simulink library "Arrowhead_Lib"  (R2026a)
settings: Solver=VariableStepAuto
undefined symbols (not defined in the file): X, Y, Z
libraries: sm_lib x17, $bdroot x3, nesl_utility x2, fl_lib x1
Description:
  | Copyright 2022-2026 The MathWorks, Inc.
settings Model: Creator=smiller  LastModifiedBy=smiller

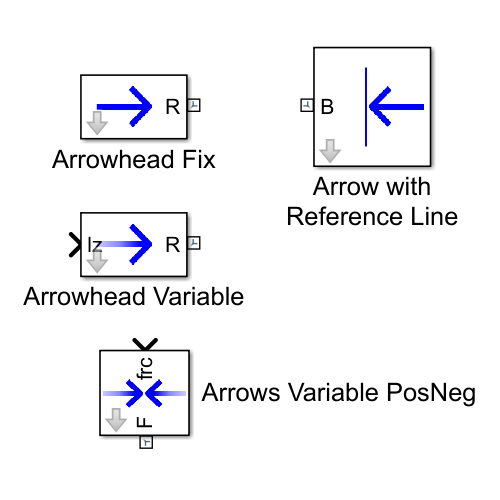
[thumbnail: Simulink's stored preview of the top-level diagram]
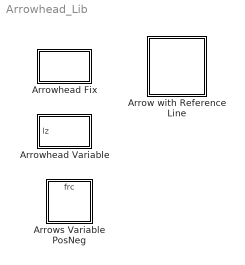
== system Arrowhead_Lib ==
  Arrow with Reference Line : Subsystem  mask{tip_l=1, tip_a=90, shaft_len=2, line_width=0.2, arrow_opc=0.5, arrow_depth=0.5, arrow_clr=[1.0 0.6 0.0], ref_ax_opc=0.5, ref_ax_offset=0.125, ref_ax_dim=[4 0.06 0.04], ref_ax_clr=[1.0 0.6 0.0]}
      mask prompts: tip_l "Tip Length (m)"; tip_a "Tip Angle (deg)"; shaft_len "Shaft Length (m)"; line_width "Line Width (m)"; arrow_opc "Arrow Opacity (0-1)"; arrow_depth "Arrow Depth (m)"; arrow_clr "Color Arrow [RGB] (0-1)"; ref_ax_opc "Opacity (0-1)"; ref_ax_offset "Offset along x (% of x length)"; ref_ax_dim "Dimensions (m)"; ref_ax_clr "Color [RGB] (0-1)"
      mask TypeOptions tip_l: Arrow/tip_l
      mask TypeOptions tip_a: Arrow/tip_a
      mask TypeOptions shaft_len: Arrow/shaft_len
      mask TypeOptions line_width: Arrow/line_width
      mask TypeOptions arrow_opc: Arrow/arrow_opc
      mask TypeOptions arrow_depth: Arrow/arrow_depth
      mask TypeOptions arrow_clr: Arrow/arrow_clr
      mask TypeOptions ref_ax_opc:
      | Reference
      | Axis/ref_ax_opc
      mask TypeOptions ref_ax_offset:
      | Reference
      | Axis/ref_ax_offset
      mask TypeOptions ref_ax_dim:
      | Reference
      | Axis/ref_ax_dim
      mask TypeOptions ref_ax_clr:
      | Reference
      | Axis/ref_ax_clr
      mask DialogControl Container4 Prompt: Arrow
      mask DialogControl Container3 Prompt: Reference Line
      mask Display: image('Arrow_with_Reference_Line_IMAGE.png')
  Arrowhead Fix : Subsystem  mask{shaft_len=2, tip_l=1, tip_a=90, arrow_clr=[0.3922 0.8314 0.07451], arrow_opc=1, arrow_depth=0.5, line_width=0.2}
      mask prompts: shaft_len "Shaft Length (m)"; tip_l "Tip Length (m)"; tip_a "Tip Angle (deg)"; arrow_clr "Color Arrow [RGB] (0-1)"; arrow_opc "Arrow Opacity (0-1)"; arrow_depth "Arrow Depth (m)"; line_width "Line Width (m)"
      mask Display: image('Arrowhead_Fix_IMAGE.png')
  Arrowhead Variable : Subsystem  mask{tip_l=1, tip_a=90, line_width=0.2, arrow_depth=0.5, arrow_clr=[0.3922 0.8314 0.07451], arrow_opc=1}
      mask prompts: tip_l "Tip Length (m)"; tip_a "Tip Angle (deg)"; line_width "Line Width (m)"; arrow_depth "Line Depth (m)"; arrow_clr "Arrow Color [RGB] (0-1)"; arrow_opc "Arrow Opacity (0-1)"
      mask Display: image('Arrowhead_Variable_IMAGE.png')
  Arrows Variable PosNeg : Subsystem  mask{max_force=4e5, max_length=10, arrow_clr=[0.3922 0.8314 0.07451], arrow_depth=0.5, line_width=0.2, tip_a=90, tip_l=1, arrow_opc=0.5}
      mask prompts: max_force "Max Force (N)"; max_length "Max Length (m)"; arrow_clr "Color Arrow [RGB] (0-1)"; arrow_depth "Arrow Depth (m)"; line_width "Line Width (m)"; tip_a "Tip Angle (deg)"; tip_l "Tip Length (m)"; arrow_opc "Arrow Opacity (0-1)"
      mask TypeOptions arrow_clr: Arrowhead Neg/arrow_clr | Arrowhead Pos/arrow_clr
      mask TypeOptions arrow_depth: Arrowhead Neg/arrow_depth | Arrowhead Pos/arrow_depth
      mask TypeOptions line_width: Arrowhead Neg/line_width | Arrowhead Pos/line_width
      mask TypeOptions tip_a: Arrowhead Neg/tip_a | Arrowhead Pos/tip_a
      mask TypeOptions tip_l: Arrowhead Neg/tip_l | Arrowhead Pos/tip_l
      mask TypeOptions arrow_opc: Arrowhead Neg/arrow_opc | Arrowhead Pos/arrow_opc
      mask Display: image('Arrows_Variable_PosNeg_IMAGE.png')

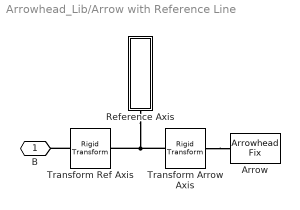
== system Arrowhead_Lib/Arrow with Reference Line ==
  Arrow : $bdroot/Arrowhead Fix  shaft_len=shaft_len  tip_l=tip_l  tip_a=tip_a  arrow_clr=arrow_clr  arrow_opc=arrow_opc  arrow_depth=arrow_depth  line_width=line_width
  Reference Axis : Subsystem  mask{ref_ax_dim=ref_ax_dim, ref_ax_offset=ref_ax_offset, ref_ax_clr=ref_ax_clr, ref_ax_opc=ref_ax_opc}
      mask prompts: ref_ax_dim "Dimensions (m)"; ref_ax_offset "Offset along x (% of x length)"; ref_ax_clr "Color [RGB] (0-1)"; ref_ax_opc "Opacity (0-1)"
  Transform Arrow Axis : sm_lib/Frames and Transforms/Rigid Transform  RotationMethod=RotationSequence  FollAlignAxisA=+X  BaseAlignAxisA=+Y  FollAlignAxisB=+Y  BaseAlignAxisB=+Z  RotationStandardAxis=+X  RotationAngle=-90  RotationAngleUnits=deg  RotationArbitraryAxis=[0 0 1]  RotationSequenceAxes=FollowerAxes  RotationSequence=XYZ  RotationSequenceAngles=[90 0 90]  RotationSequenceAnglesUnits=deg  RotationMatrix=[1 0 0; 0 1 0; 0 0 1]  Quaternion=[1 0 0 0]  TranslationMethod=None  TranslationCartesianOffset=[0 0 0]  TranslationCartesianOffsetUnits=m  TranslationStandardAxis=+Z  TranslationStandardOffset=0  TranslationStandardOffsetUnits=m  TranslationROffset=0  TranslationROffsetUnits=m  TranslationThetaOffset=0  TranslationThetaOffsetUnits=deg  TranslationZOffset=0  TranslationZOffsetUnits=m
  Transform Ref Axis : sm_lib/Frames and Transforms/Rigid Transform  RotationMethod=StandardAxis  FollAlignAxisA=+X  BaseAlignAxisA=+Y  FollAlignAxisB=+Y  BaseAlignAxisB=+Z  RotationStandardAxis=+Z  RotationAngle=90  RotationAngleUnits=deg  RotationArbitraryAxis=[0 0 1]  RotationSequenceAxes=FollowerAxes  RotationSequence=XYZ  RotationSequenceAngles=[90 0 90]  RotationSequenceAnglesUnits=deg  RotationMatrix=[1 0 0; 0 1 0; 0 0 1]  Quaternion=[1 0 0 0]  TranslationMethod=None  TranslationCartesianOffset=[0 0 0]  TranslationCartesianOffsetUnits=m  TranslationStandardAxis=+Z  TranslationStandardOffset=0  TranslationStandardOffsetUnits=m  TranslationROffset=0  TranslationROffsetUnits=m  TranslationThetaOffset=0  TranslationThetaOffsetUnits=deg  TranslationZOffset=0  TranslationZOffsetUnits=m
  B : PMIOPort  Side=Left
  connections:
  Transform Arrow Axis/RConn1 -- Arrow/RConn1
  Transform Arrow Axis/LConn1 -- Reference Axis/LConn1 -- Transform Ref Axis/RConn1
  Transform Ref Axis/LConn1 -- B/RConn1

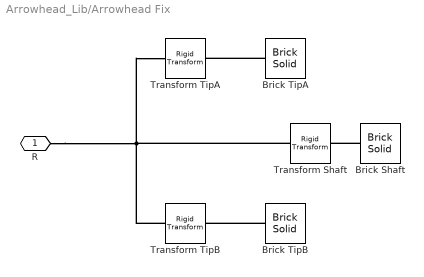
== system Arrowhead_Lib/Arrowhead Fix ==
  Brick Shaft : sm_lib/Body Elements/Brick Solid  BrickDimensions=[arrow_depth line_width shaft_len]  BrickDimensionsUnits=m  ExportEntireGeometry=off  InertiaType=PointMass  BasedOnType=Density  Density=1000  DensityUnits=kg/m^3  Mass=1e-3  MassUnits=kg  CenterOfMass=[0 0 0]  CenterOfMassUnits=m  MomentsOfInertia=[1 1 1]  MomentsOfInertiaUnits=kg*m^2  ProductsOfInertia=[0 0 0]  ProductsOfInertiaUnits=kg*m^2  GraphicType=FromGeometry  MarkerShape=Sphere  MarkerSize=10  GraphicVisPropType=AdvancedVisualProperties  GraphicDiffuseColor=[arrow_clr arrow_opc]  GraphicOpacity=1.0  GraphicSpecularColor=[0.5 0.5 0.5 arrow_opc]  GraphicAmbientColor=[0.15 0.15 0.15 arrow_opc]  GraphicEmissiveColor=[arrow_clr*0.3 arrow_opc]  GraphicShininess=75  DoExposeReferenceFrame=off  SerializedFrames=<Frames><Frame><Id>Frame1</Id><Value><Name>B</Name><Origin><Source>GeometricFeature</Source><FeatureName>-z surface</FeatureName></Origin><PrimaryAxis><DefinedDirection>+Z</DefinedDirection><Source>ReferenceFrame</Source><SourceDirection>+Z</SourceDirection><FeatureName></FeatureName></PrimaryAxis><SecondaryAxis><DefinedDirection>+X</DefinedDirection><Source>ReferenceFrame</Source><SourceDirection>+X</SourceDirection><FeatureName></FeatureName></SecondaryAxis></Value></Frame></Frames>
  Brick TipA : sm_lib/Body Elements/Brick Solid  BrickDimensions=[arrow_depth line_width tip_l]  BrickDimensionsUnits=m  ExportEntireGeometry=off  InertiaType=PointMass  BasedOnType=Mass  Density=1000  DensityUnits=kg/m^3  Mass=1e-3  MassUnits=kg  CenterOfMass=[0 0 0]  CenterOfMassUnits=m  MomentsOfInertia=[1 1 1]  MomentsOfInertiaUnits=kg*m^2  ProductsOfInertia=[0 0 0]  ProductsOfInertiaUnits=kg*m^2  GraphicType=FromGeometry  MarkerShape=Sphere  MarkerSize=10  GraphicVisPropType=AdvancedVisualProperties  GraphicDiffuseColor=[arrow_clr arrow_opc]  GraphicOpacity=1.0  GraphicSpecularColor=[0.5 0.5 0.5 arrow_opc]  GraphicAmbientColor=[0.15 0.15 0.15 arrow_opc]  GraphicEmissiveColor=[arrow_clr*0.3 arrow_opc]  GraphicShininess=75  DoExposeReferenceFrame=off  SerializedFrames=<Frames><Frame><Id>Frame1</Id><Value><Name>B</Name><Origin><Source>GeometricFeature</Source><FeatureName>-z surface</FeatureName></Origin><PrimaryAxis><DefinedDirection>+Z</DefinedDirection><Source>ReferenceFrame</Source><SourceDirection>+Z</SourceDirection><FeatureName></FeatureName></PrimaryAxis><SecondaryAxis><DefinedDirection>+X</DefinedDirection><Source>ReferenceFrame</Source><SourceDirection>+X</SourceDirection><FeatureName></FeatureName></SecondaryAxis></Value></Frame></Frames>
  Brick TipB : sm_lib/Body Elements/Brick Solid  BrickDimensions=[arrow_depth line_width tip_l]  BrickDimensionsUnits=m  ExportEntireGeometry=off  InertiaType=PointMass  BasedOnType=Density  Density=1000  DensityUnits=kg/m^3  Mass=1e-3  MassUnits=kg  CenterOfMass=[0 0 0]  CenterOfMassUnits=m  MomentsOfInertia=[1 1 1]  MomentsOfInertiaUnits=kg*m^2  ProductsOfInertia=[0 0 0]  ProductsOfInertiaUnits=kg*m^2  GraphicType=FromGeometry  MarkerShape=Sphere  MarkerSize=10  GraphicVisPropType=AdvancedVisualProperties  GraphicDiffuseColor=[arrow_clr arrow_opc]  GraphicOpacity=1.0  GraphicSpecularColor=[0.5 0.5 0.5 arrow_opc]  GraphicAmbientColor=[0.15 0.15 0.15 arrow_opc]  GraphicEmissiveColor=[arrow_clr*0.3 arrow_opc]  GraphicShininess=75  DoExposeReferenceFrame=off  SerializedFrames=<Frames><Frame><Id>Frame1</Id><Value><Name>B</Name><Origin><Source>GeometricFeature</Source><FeatureName>-z surface</FeatureName></Origin><PrimaryAxis><DefinedDirection>+Z</DefinedDirection><Source>ReferenceFrame</Source><SourceDirection>+Z</SourceDirection><FeatureName></FeatureName></PrimaryAxis><SecondaryAxis><DefinedDirection>+X</DefinedDirection><Source>ReferenceFrame</Source><SourceDirection>+X</SourceDirection><FeatureName></FeatureName></SecondaryAxis></Value></Frame></Frames>
  Transform Shaft : sm_lib/Frames and Transforms/Rigid Transform  RotationMethod=None  FollAlignAxisA=+X  BaseAlignAxisA=+Y  FollAlignAxisB=+Y  BaseAlignAxisB=+Z  RotationStandardAxis=+Z  RotationAngle=0.0  RotationAngleUnits=deg  RotationArbitraryAxis=[0 0 1]  RotationSequenceAxes=FollowerAxes  RotationSequence=XYX  RotationSequenceAngles=[0 0 0]  RotationSequenceAnglesUnits=deg  RotationMatrix=[1 0 0; 0 1 0; 0 0 1]  Quaternion=[1 0 0 0]  TranslationMethod=StandardAxis  TranslationCartesianOffset=[0 0 0]  TranslationCartesianOffsetUnits=m  TranslationStandardAxis=+Z  TranslationStandardOffset=(line_width/2)/tand(tip_a/2)  TranslationStandardOffsetUnits=m  TranslationROffset=0  TranslationROffsetUnits=m  TranslationThetaOffset=0  TranslationThetaOffsetUnits=deg  TranslationZOffset=0  TranslationZOffsetUnits=m
  Transform TipA : sm_lib/Frames and Transforms/Rigid Transform  RotationMethod=StandardAxis  FollAlignAxisA=+X  BaseAlignAxisA=+Y  FollAlignAxisB=+Y  BaseAlignAxisB=+Z  RotationStandardAxis=+X  RotationAngle=tip_a/2  RotationAngleUnits=deg  RotationArbitraryAxis=[0 0 1]  RotationSequenceAxes=FollowerAxes  RotationSequence=XYX  RotationSequenceAngles=[0 0 0]  RotationSequenceAnglesUnits=deg  RotationMatrix=[1 0 0; 0 1 0; 0 0 1]  Quaternion=[1 0 0 0]  TranslationMethod=Cartesian  TranslationCartesianOffset=[0 0 0]*tip_l/2*sind(tip_a/2)+[0 1 1]*line_width/2*sind(tip_a/2)  TranslationCartesianOffsetUnits=m  TranslationStandardAxis=+Y  TranslationStandardOffset=tip_l/2*sind(tip_a/2)  TranslationStandardOffsetUnits=m  TranslationROffset=0  TranslationROffsetUnits=m  TranslationThetaOffset=0  TranslationThetaOffsetUnits=deg  TranslationZOffset=0  TranslationZOffsetUnits=m
  Transform TipB : sm_lib/Frames and Transforms/Rigid Transform  RotationMethod=StandardAxis  FollAlignAxisA=+X  BaseAlignAxisA=+Y  FollAlignAxisB=+Y  BaseAlignAxisB=+Z  RotationStandardAxis=-X  RotationAngle=tip_a/2  RotationAngleUnits=deg  RotationArbitraryAxis=[0 0 1]  RotationSequenceAxes=FollowerAxes  RotationSequence=XYX  RotationSequenceAngles=[0 0 0]  RotationSequenceAnglesUnits=deg  RotationMatrix=[1 0 0; 0 1 0; 0 0 1]  Quaternion=[1 0 0 0]  TranslationMethod=Cartesian  TranslationCartesianOffset=[0 0 0]*tip_l/2*sind(tip_a/2)+[0 -1 1]*line_width/2*sind(tip_a/2)  TranslationCartesianOffsetUnits=m  TranslationStandardAxis=+Y  TranslationStandardOffset=tip_l/2*sind(tip_a/2)  TranslationStandardOffsetUnits=m  TranslationROffset=0  TranslationROffsetUnits=m  TranslationThetaOffset=0  TranslationThetaOffsetUnits=deg  TranslationZOffset=0  TranslationZOffsetUnits=m
  R : PMIOPort  Side=Right
  connections:
  Brick Shaft/LConn1 -- Transform Shaft/RConn1
  Brick TipB/LConn1 -- Transform TipB/RConn1
  Transform TipB/LConn1 -- Transform Shaft/LConn1 -- Transform TipA/LConn1 -- R/RConn1
  Brick TipA/LConn1 -- Transform TipA/RConn1

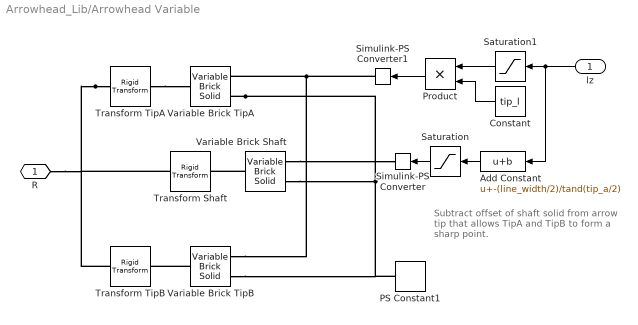
== system Arrowhead_Lib/Arrowhead Variable ==
  note: Subtract offset of shaft solid from arrow tip that allows TipA and TipB to form a sharp point.
  lz : Inport
  Add Constant : Bias  Bias=-(line_width/2)/tand(tip_a/2)  SaturateOnIntegerOverflow=off
  Constant : Constant  Value=tip_l
  PS Constant1 : fl_lib/Physical Signals/Sources/PS Constant  constant=1e-3 kg
  Product : Product
  Saturation : Saturate  UpperLimit=Inf  LowerLimit=1e-3  ZeroCross=off
  Saturation1 : Saturate  UpperLimit=1  LowerLimit=1e-3  ZeroCross=off
  Simulink-PS Converter : nesl_utility/Simulink-PS Converter  PhysicalDomain=network_engine_domain  SubClassName=ps_input  LeftPortType=input  RightPortType=output  PseudoPeriodic=off  Frequencies=[]  NoiseDistribution=none  NoiseParameters=[]  Unit=1  AffineConversion=off  FilteringAndDerivatives=provide  SimscapeFilterOrder=1  InputFilterTimeConstant=0.001  UdotUserProvided=0
  Simulink-PS Converter1 : nesl_utility/Simulink-PS Converter  PhysicalDomain=network_engine_domain  SubClassName=ps_input  LeftPortType=input  RightPortType=output  PseudoPeriodic=off  Frequencies=[]  NoiseDistribution=none  NoiseParameters=[]  Unit=1  AffineConversion=off  FilteringAndDerivatives=provide  SimscapeFilterOrder=1  InputFilterTimeConstant=0.001  UdotUserProvided=0
  Transform Shaft : sm_lib/Frames and Transforms/Rigid Transform  RotationMethod=None  FollAlignAxisA=+X  BaseAlignAxisA=+Y  FollAlignAxisB=+Y  BaseAlignAxisB=+Z  RotationStandardAxis=+Z  RotationAngle=0.0  RotationAngleUnits=deg  RotationArbitraryAxis=[0 0 1]  RotationSequenceAxes=FollowerAxes  RotationSequence=XYX  RotationSequenceAngles=[0 0 0]  RotationSequenceAnglesUnits=deg  RotationMatrix=[1 0 0; 0 1 0; 0 0 1]  Quaternion=[1 0 0 0]  TranslationMethod=StandardAxis  TranslationCartesianOffset=[0 0 0]  TranslationCartesianOffsetUnits=m  TranslationStandardAxis=+Z  TranslationStandardOffset=(line_width/2)/tand(tip_a/2)  TranslationStandardOffsetUnits=m  TranslationROffset=0  TranslationROffsetUnits=m  TranslationThetaOffset=0  TranslationThetaOffsetUnits=deg  TranslationZOffset=0  TranslationZOffsetUnits=m
  Transform TipA : sm_lib/Frames and Transforms/Rigid Transform  RotationMethod=StandardAxis  FollAlignAxisA=+X  BaseAlignAxisA=+Y  FollAlignAxisB=+Y  BaseAlignAxisB=+Z  RotationStandardAxis=+X  RotationAngle=tip_a/2  RotationAngleUnits=deg  RotationArbitraryAxis=[0 0 1]  RotationSequenceAxes=FollowerAxes  RotationSequence=XYX  RotationSequenceAngles=[0 0 0]  RotationSequenceAnglesUnits=deg  RotationMatrix=[1 0 0; 0 1 0; 0 0 1]  Quaternion=[1 0 0 0]  TranslationMethod=Cartesian  TranslationCartesianOffset=[0 0 0]*tip_l/2*sind(tip_a/2)+[0 1 1]*line_width/2*sind(tip_a/2)  TranslationCartesianOffsetUnits=m  TranslationStandardAxis=+Y  TranslationStandardOffset=tip_l/2*sind(tip_a/2)  TranslationStandardOffsetUnits=m  TranslationROffset=0  TranslationROffsetUnits=m  TranslationThetaOffset=0  TranslationThetaOffsetUnits=deg  TranslationZOffset=0  TranslationZOffsetUnits=m
  Transform TipB : sm_lib/Frames and Transforms/Rigid Transform  RotationMethod=StandardAxis  FollAlignAxisA=+X  BaseAlignAxisA=+Y  FollAlignAxisB=+Y  BaseAlignAxisB=+Z  RotationStandardAxis=-X  RotationAngle=tip_a/2  RotationAngleUnits=deg  RotationArbitraryAxis=[0 0 1]  RotationSequenceAxes=FollowerAxes  RotationSequence=XYX  RotationSequenceAngles=[0 0 0]  RotationSequenceAnglesUnits=deg  RotationMatrix=[1 0 0; 0 1 0; 0 0 1]  Quaternion=[1 0 0 0]  TranslationMethod=Cartesian  TranslationCartesianOffset=[0 0 0]*tip_l/2*sind(tip_a/2)+[0 -1 1]*line_width/2*sind(tip_a/2)  TranslationCartesianOffsetUnits=m  TranslationStandardAxis=+Y  TranslationStandardOffset=tip_l/2*sind(tip_a/2)  TranslationStandardOffsetUnits=m  TranslationROffset=0  TranslationROffsetUnits=m  TranslationThetaOffset=0  TranslationThetaOffsetUnits=deg  TranslationZOffset=0  TranslationZOffsetUnits=m
  Variable Brick Shaft : sm_lib/Body Elements/Variable Mass/Variable Brick Solid  ComputedVariable=Density  XLengthType=Constant  XLength=arrow_depth  XLengthUnits=m  YLengthType=Constant  YLength=line_width  YLengthUnits=m  ZLengthType=ProvidedByInput  ZLength=0.5  ZLengthUnits=m  DensityType=Constant  Density=1000  DensityUnits=kg/m^3  MassType=ProvidedByInput  Mass=1  MassUnits=kg  SenseXLength=off  SenseYLength=off  SenseZLength=off  SenseDensity=off  SenseMass=off  SenseCenterOfMass=off  SenseInertiaMatrix=off  GraphicType=FromGeometry  MarkerShape=Sphere  MarkerSize=10  GraphicVisPropType=AdvancedVisualProperties  GraphicDiffuseColor=[arrow_clr arrow_opc]  GraphicOpacity=1.0  GraphicSpecularColor=[0.5 0.5 0.5 arrow_opc]  GraphicAmbientColor=[0.15 0.15 0.15 arrow_opc]  GraphicEmissiveColor=[arrow_clr*0.3 arrow_opc]  GraphicShininess=75
  Variable Brick TipA : sm_lib/Body Elements/Variable Mass/Variable Brick Solid  ComputedVariable=Density  XLengthType=Constant  XLength=arrow_depth  XLengthUnits=m  YLengthType=Constant  YLength=line_width  YLengthUnits=m  ZLengthType=ProvidedByInput  ZLength=0.5  ZLengthUnits=m  DensityType=Constant  Density=1000  DensityUnits=kg/m^3  MassType=ProvidedByInput  Mass=1  MassUnits=kg  SenseXLength=off  SenseYLength=off  SenseZLength=off  SenseDensity=off  SenseMass=off  SenseCenterOfMass=off  SenseInertiaMatrix=off  GraphicType=FromGeometry  MarkerShape=Sphere  MarkerSize=10  GraphicVisPropType=AdvancedVisualProperties  GraphicDiffuseColor=[arrow_clr arrow_opc]  GraphicOpacity=1.0  GraphicSpecularColor=[0.5 0.5 0.5 arrow_opc]  GraphicAmbientColor=[0.15 0.15 0.15 arrow_opc]  GraphicEmissiveColor=[arrow_clr*0.3 arrow_opc]  GraphicShininess=75
  Variable Brick TipB : sm_lib/Body Elements/Variable Mass/Variable Brick Solid  ComputedVariable=Density  XLengthType=Constant  XLength=arrow_depth  XLengthUnits=m  YLengthType=Constant  YLength=line_width  YLengthUnits=m  ZLengthType=ProvidedByInput  ZLength=0.5  ZLengthUnits=m  DensityType=Constant  Density=1000  DensityUnits=kg/m^3  MassType=ProvidedByInput  Mass=1  MassUnits=kg  SenseXLength=off  SenseYLength=off  SenseZLength=off  SenseDensity=off  SenseMass=off  SenseCenterOfMass=off  SenseInertiaMatrix=off  GraphicType=FromGeometry  MarkerShape=Sphere  MarkerSize=10  GraphicVisPropType=AdvancedVisualProperties  GraphicDiffuseColor=[arrow_clr arrow_opc]  GraphicOpacity=1.0  GraphicSpecularColor=[0.5 0.5 0.5 arrow_opc]  GraphicAmbientColor=[0.15 0.15 0.15 arrow_opc]  GraphicEmissiveColor=[arrow_clr*0.3 arrow_opc]  GraphicShininess=75
  R : PMIOPort  Side=Right
  wires:
  lz/1 -> Add Constant/1, Saturation1/1
  Saturation/1 -> Simulink-PS Converter/1
  Saturation1/1 -> Product/1
  Constant/1 -> Product/2
  Product/1 -> Simulink-PS Converter1/1
  Add Constant/1 -> Saturation/1
  connections:
  Variable Brick Shaft/RConn1 -- Transform Shaft/RConn1
  Variable Brick TipB/RConn1 -- Transform TipB/RConn1
  Transform TipA/LConn1 -- R/RConn1 -- Transform TipB/LConn1 -- Transform Shaft/LConn1
  Variable Brick TipA/LConn2 -- Variable Brick Shaft/LConn2 -- Variable Brick TipB/LConn2 -- PS Constant1/RConn1
  Transform TipA/RConn1 -- Variable Brick TipA/RConn1
  Simulink-PS Converter1/RConn1 -- Variable Brick TipB/LConn1 -- Variable Brick TipA/LConn1
  Variable Brick Shaft/LConn1 -- Simulink-PS Converter/RConn1

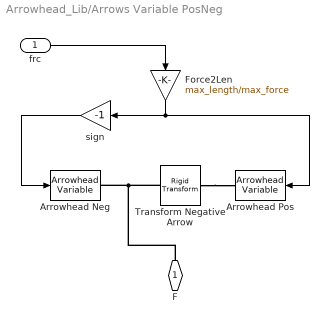
== system Arrowhead_Lib/Arrows Variable PosNeg ==
  frc : Inport
  Arrowhead Neg : $bdroot/Arrowhead Variable  tip_l=tip_l  tip_a=tip_a  line_width=line_width  arrow_depth=arrow_depth  arrow_clr=arrow_clr  arrow_opc=arrow_opc
  Arrowhead Pos : $bdroot/Arrowhead Variable  tip_l=tip_l  tip_a=tip_a  line_width=line_width  arrow_depth=arrow_depth  arrow_clr=arrow_clr  arrow_opc=arrow_opc
  Force2Len : Gain  Gain=max_length/max_force
  Transform Negative Arrow : sm_lib/Frames and Transforms/Rigid Transform  RotationMethod=StandardAxis  FollAlignAxisA=+X  BaseAlignAxisA=+Y  FollAlignAxisB=+Y  BaseAlignAxisB=+Z  RotationStandardAxis=+X  RotationAngle=180  RotationAngleUnits=deg  RotationArbitraryAxis=[0 0 1]  RotationSequenceAxes=FollowerAxes  RotationSequence=XYX  RotationSequenceAngles=[0 0 0]  RotationSequenceAnglesUnits=deg  RotationMatrix=[1 0 0; 0 1 0; 0 0 1]  Quaternion=[1 0 0 0]  TranslationMethod=None  TranslationCartesianOffset=[0 0 0]  TranslationCartesianOffsetUnits=m  TranslationStandardAxis=+Z  TranslationStandardOffset=0  TranslationStandardOffsetUnits=m  TranslationROffset=0  TranslationROffsetUnits=m  TranslationThetaOffset=0  TranslationThetaOffsetUnits=deg  TranslationZOffset=0  TranslationZOffsetUnits=m
  sign : Gain  Gain=-1
  F : PMIOPort  Side=Right
  wires:
  frc/1 -> Force2Len/1
  Force2Len/1 -> Arrowhead Pos/1, sign/1
  sign/1 -> Arrowhead Neg/1
  connections:
  Transform Negative Arrow/RConn1 -- Arrowhead Pos/RConn1
  Transform Negative Arrow/LConn1 -- F/RConn1 -- Arrowhead Neg/RConn1

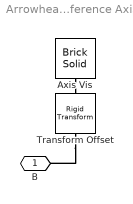
== system Arrowhead_Lib/Arrow with Reference Line/Reference Axis ==
  Axis Vis : sm_lib/Body Elements/Brick Solid  BrickDimensions=ref_ax_dim  BrickDimensionsUnits=m  ExportEntireGeometry=off  InertiaType=CalculateFromGeometry  BasedOnType=Density  Density=1  DensityUnits=kg/m^3  Mass=1  MassUnits=kg  CenterOfMass=[0 0 0]  CenterOfMassUnits=m  MomentsOfInertia=[1 1 1]  MomentsOfInertiaUnits=kg*m^2  ProductsOfInertia=[0 0 0]  ProductsOfInertiaUnits=kg*m^2  GraphicType=FromGeometry  MarkerShape=Sphere  MarkerSize=10  GraphicVisPropType=SimpleVisualProperties  GraphicDiffuseColor=ref_ax_clr  GraphicOpacity=ref_ax_opc  GraphicSpecularColor=[0.5 0.5 0.5 1.0]  GraphicAmbientColor=[0.15 0.15 0.15 1.0]  GraphicEmissiveColor=[0.0 0.0 0.0 1.0]  GraphicShininess=75  DoExposeReferenceFrame=on  SerializedFrames=<Frames/>
  Transform Offset : sm_lib/Frames and Transforms/Rigid Transform  RotationMethod=None  FollAlignAxisA=+X  BaseAlignAxisA=+Y  FollAlignAxisB=+Y  BaseAlignAxisB=+Z  RotationStandardAxis=+Z  RotationAngle=0.0  RotationAngleUnits=deg  RotationArbitraryAxis=[0 0 1]  RotationSequenceAxes=FollowerAxes  RotationSequence=XYX  RotationSequenceAngles=[0 0 0]  RotationSequenceAnglesUnits=deg  RotationMatrix=[1 0 0; 0 1 0; 0 0 1]  Quaternion=[1 0 0 0]  TranslationMethod=StandardAxis  TranslationCartesianOffset=[0 0 0]  TranslationCartesianOffsetUnits=m  TranslationStandardAxis=+X  TranslationStandardOffset=ref_ax_dim(1)*ref_ax_offset  TranslationStandardOffsetUnits=m  TranslationROffset=0  TranslationROffsetUnits=m  TranslationThetaOffset=0  TranslationThetaOffsetUnits=deg  TranslationZOffset=0  TranslationZOffsetUnits=m
  B : PMIOPort  Side=Left
  connections:
  Axis Vis/RConn1 -- Transform Offset/RConn1
  Transform Offset/LConn1 -- B/RConn1
